simulink model "uc3_preparation1_2017"  (R2018a)
settings: Solver=FixedStepDiscrete  StartTime=0.0  StopTime=0.6  FixedStep=2e-5  RelTol=1e-3
libraries: simulink x10, hdlsllib x10, dspswit3 x1
(part 2 of 2)

== system uc3_preparation1_2017/CandHDL_hdl/hdlgenerate/Subsystem/Dynamic_Calculations/FPGA_Calculation/Write_to_Memory ==
  note: WRITE TO MEMORY BLOCK
  readAddr : Inport
  c0 : Inport  Port=2
  c1 : Inport  Port=3
  c2 : Inport  Port=4
  write : Inport  Port=5
  writeAddr : Inport  Port=6
  Single Port RAM : hdlsllib/HDL RAMs/Single Port RAM  ram_size=8  dout_type=New data
      settings: SourceProductName=HDL Coder  SourceProductBaseCode=HD
  Single Port RAM1 : hdlsllib/HDL RAMs/Single Port RAM  ram_size=8  dout_type=New data
      settings: SourceProductName=HDL Coder  SourceProductBaseCode=HD
  Single Port RAM2 : hdlsllib/HDL RAMs/Single Port RAM  ram_size=8  dout_type=New data
      settings: SourceProductName=HDL Coder  SourceProductBaseCode=HD
  Switch : Switch  Criteria=u2 > Threshold
  c0Ram : Outport
  c1Ram : Outport  Port=2
  c2Ram : Outport  Port=3
  wires:
  Single Port RAM/1 -> c0Ram/1
  Switch/1 -> Single Port RAM/2, Single Port RAM2/2, Single Port RAM1/2
  [wr] -> Single Port RAM/3
  write/1 -> [wr], Switch/2
  writeAddr/1 -> Switch/1
  readAddr/1 -> Switch/3
  [wr] -> Single Port RAM1/3
  [wr] -> Single Port RAM2/3
  Single Port RAM1/1 -> c1Ram/1
  Single Port RAM2/1 -> c2Ram/1
  c0/1 -> Single Port RAM/1
  c1/1 -> Single Port RAM1/1
  c2/1 -> Single Port RAM2/1

== system uc3_preparation1_2017/CandHDL_hdl/hdlgenerate/Subsystem/Dynamic_Calculations/FPGA_Calculation/Polynomial_Calculation/Difference_Time ==
  note: Time Difference (x - x0)
  Time : Inport
  breakpoints : Inport  Port=2
  Add : Sum  Inputs=+-  OutDataTypeStr=fixdt(1,27,19)
  Delay : Delay  DelayLength=1
  Detect Change : simulink/Logic and Bit Operations/Detect Change  vinit=0  OutDataTypeStr=boolean
  Switch : Switch  Criteria=u2 > Threshold
  dt : Outport
  wires:
  Switch/1 -> Delay/1, Add/2
  Time/1 -> Switch/1, Add/1
  breakpoints/1 -> Detect Change/1
  Delay/1 -> Switch/3
  Detect Change/1 -> Switch/2
  Add/1 -> dt/1

== stateflow chart uc3_preparation1_2017/CandHDL_c/cgenerate/Subsystem/Counter/Chart ==
  settings: executeAtInitialization=1
  state sate2
    entry:
    strobe_temp=0;
    during:
    counter=0;
  state state1
    entry:
    strobe_temp=strobe;
    counter=0;
    during :
    counter=counter+1;
  (default) -> state1
  state1 -> sate2 : [(counter >128)]
  sate2 -> state1 : [(strobe==1)]
  data: strobe input single; counter output single; strobe_temp local single

== matlab function uc3_preparation1_2017/CandHDL_c/cgenerate/Static Calculations/RT_CPU ==
  data: ch input; A input [0..1]; mode input [0..2]; dutyCycle input [0..1]; breakPoints input [4..255]; pOrder input [0..3]; f input [0..10000]; cc output size=[256 4]; b output size=[1 255] [4..255]; rst output
function [cc,b,rst]  = fcn(ch,A,mode,dutyCycle, breakPoints,pOrder, f)
%% RT CPU
%   This Embedded Matlab function calculates the polynomial coefficients
%       and breaks points according to the external user settings. 
%       Three different waveforms can be selected with "mode"
%               0: Sine
%               1: Rectangular (not implemented yet)
%               2: Triangular  (not implemented yet)
%       
%    Author: R. Estrada, FH JOANNEUM, 2018
%
%%
    % Declaration of global variables
    persistent cc0 b0 i0;
    rst = single(0);
    if isempty(cc0)    
        cc0 = single(zeros(101,3));
        b0  = single(zeros(1,101));
        i0  = single(0);  %Used to checks if the program is running for the 1st time
    end
    
    
    if (ch || i0<1)        
        
        rst = single(1);
        i0=single(1);
        ch = 0;
        
        %Bound values of breakpoints
        assert(breakPoints<=256);
        
        cc = single(zeros(breakPoints+1,3));        %% Creates coefficients array 
        b  = single(zeros(1,(breakPoints + 1)));    %% Create breakpoints array 
        tf = single(1/f);
        y  = single(zeros(1 , (breakPoints + 1)));
        x= single(linspace(0,1,breakPoints+1));
        x1= single(linspace(0,1,breakPoints));
        
        switch mode
            case 0 % Sine wave
                                
                y  = A*sin(2*pi.*x);   
            
            case 1 % Square Wave  
                
                y = (x < dutyCycle).*(A) + (x >= dutyCycle).*(-A);
                y(breakPoints+1) = A;
                    
            case 2 % Triangular wave                
                
                if (dutyCycle ==0 || dutyCycle == 1)     %To avoid division by 0
                    
                    y = (dutyCycle == 1).*(-A+(x1*A*2)) +...
                        (dutyCycle ==0).*(-A+((1-x1)*A*2));
                    y= [y y(1)];
                else
                    
                    y = (x <= dutyCycle).*(-A+(x*A*(2/dutyCycle)))+...
                        (x > dutyCycle).*(-A+((1-x)*A*(2/(1-dutyCycle))));

                end
               
            otherwise
                y  = single(0);
        end

        %% Finite difference
        %   Coefficients
        cfd = [  1 0 0 0;...
                -1 1 0 0; ...
                 1 -2 1 0; ...
                -1 3 -3 1];

        % Extend array around the end
        yy = [y y(2:4)];
        
        for j=0:1:breakPoints                        % Sweep of break points
            b(1,j+1)=j*tf/breakPoints;               % Store actual break point
            ys = [yy(j+1) yy(j+2) yy(j+3) yy(j+4)];   % Prepare y vector
            for i=0:1:pOrder       
                dy = cfd(i+1,:) * ys'/(tf/breakPoints)^i; % Compute pOrder derivate        
                cc(j+1,i+1)= dy/factorial(i);        
            end                  
        end
        
        % Store values in global variables
        cc0 = cc;  
        b0  = b;
    else
        % Keep the previous values
        cc = cc0;
        b  = b0;
    end %end of main if
    
end % Function

== matlab function uc3_preparation1_2017/CandHDL_c/cgenerate/Subsystem/RT_CPU ==
  data: A input [0..1]; f input; cc output; strobe output; mode input [0..2]; din input [0..100]; n input [0..3]; b output
function [cc,strobe,b]  = fcn(A,f,mode,din,n)
%% RT CPU
%   This Embedded Matlab function calculates the polynomial coefficients
%       and breaks points according to the external user settings. 
%       Three different waveforms can be selected with "mode"
%               0: Sine
%               1: Rectangular (not implemented yet)
%               2: Triangular  (not implemented yet)
%
%       
%    Author: R. Estrada, FH JOANNEUM, 2018
%
%%
    % Declaration of global variables
    persistent cc0 b0 i0 ;
    d=din
    d_sep=(din*1.28)
    % This is executed only once during Initialization
    if isempty(cc0)    
        cc0 =  single(zeros(129,3));  %    zeros(101,3);
        b0  = single(zeros(1,129)); %zeros(1,101);
        nb = single(128);
        n = single(2);
        
        cc =  single(zeros(129,3));
        b  = single(zeros(1,129));
        i0=single(0);
         
    end
    strobe=single(0);
    
    % Calculation is done only once
    %  Note: An external signal together with an OR condition can be added
    %        for recalculating the coefficients and break points on demand
    if i0<single(1)        
        i0=single(1);

         cc = single(zeros(129,3));   
         b  = single(zeros(1,129));
         nb = single(128);
         tf = single(1/f);
         
         strobe=single(1);
         assert(nb<=256);

         %d=single(1);
         
         
        switch mode
            case 0 % Sine wave
               % nb = 100;        % Number of break points
                %n  = 2;         % Polynomial order
                %y  = A*sin(2*pi*f.*linspace(0,1/f,nb+1));        
                y  = single(A*sin(2*pi*f.*linspace(0,1/f,129))); 
                
            case 1 %Rectangle wave 
               
                %assert((A>0)&&(A<=1));
               % assert(nb<=256);
                i=1;
                y=single(zeros(1,129));
             
               for j=0:tf/(128):tf
                  if  j<=tf*d
                   
                        y(i)=single(A);
                    else
                        y(i)=-single(A);
                  end
                    i=i+1;
                end
                
            case 2 %triangle wave
                
                i=1;
                  y=single(zeros(1,129));
                  for j=0:tf/(128):tf
                      if i==1
                            y(i)=single(A);
                      else
                          if j<=tf*d
                              y(i)=single(y(i-1)+2*(A/128)/(d));
                          else
                              y(i)=single(y(i-1)-2*(A/128)/(1-d));
                          end
                      end
                      i=i+1;
                  end 
            case 3
                 
                %assert((A>0)&&(A<=1));
               % assert(nb<=256);
                      y=single(zeros(1,129));
             
               for j=1:128
                  if  j<=d_sep
                   
                        y(j)=single(A);
                    else
                        y(j)=-single(A);
                  end
                    y(j+1)=A;
                    
               end
        
            case 4
                y=single(zeros(1,129));
                    for i=1:128
                        if i<=d_sep
                            y(i)=single(A-(A/d_sep));
                        else
                            y(i)=single(-1*A+(A/(128-d_sep-i)));
                        end
                         
                    end
                     y(i+1)=A;
                
              
            otherwise
                nb = single(128);
                n = single(2);
               y=single(zeros(1,129));
        end

        %% Finite difference
        %   Coefficients
        cfd = [  1 0 0 0;...
                -1 1 0 0; ...
                 1 -2 1 0; ...
                -1 3 -3 1];

        % Extend array around the end
        yy = [y y(2:4)];
        
        for j=0:1:nb                        % Sweep of break points
            b(1,j+1)=j*tf/nb;               % Store actual break point
            ys = [yy(j+1) yy(j+2) yy(j+3) yy(j+4)];   % Prepare y vector
            for i=0:1:n       
                dy = cfd(i+1,:) * ys'/(f/nb)^i; % Compute n derivate        
                cc(j+1,i+1)= dy/factorial(i);        
            end                  
        end
        
        % Store values in global variables
        cc0 = cc;  
        b0  = b;
     %   strobe0=strobe;
    else
        % Keep the previous values
        cc = cc0;
        b  = b0;
    
    end %end of main if
    
end % Function
